simulink model "PID"  (R2021b)
settings: Solver=VariableStepAuto  StartTime=0.0  StopTime=10.0  RelTol=1e-3
settings Model: Creator=Studenci  LastModifiedBy=Studenci

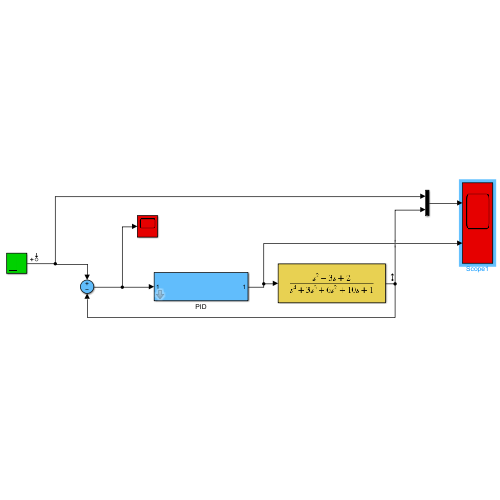
[thumbnail: Simulink's stored preview of the top-level diagram]
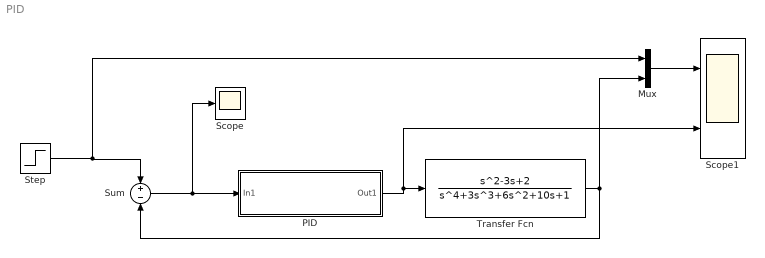
== system PID ==
  Mux : Mux  Inputs=2
  PID : Subsystem  mask{Kp=1.5288, Ki=0.4312, Kd=1.3550}
      mask prompts: Kp "Kp ="; Ki "Ki ="; Kd "Kd ="
  Scope : Scope
  Scope1 : Scope  NumInputPorts=2
  Step : Step  Time=0  SampleTime=0
  Sum : Sum  Inputs=+-
  Transfer Fcn : TransferFcn  Numerator=[1 -3 2]  Denominator=[1 3 6 10 1]
  wires:
  Step/1 -> Sum/1, Mux/1
  Sum/1 -> Scope/1, PID/1(In1)
  Mux/1 -> Scope1/1
  PID/1(Out1) -> Scope1/2, Transfer Fcn/1
  Transfer Fcn/1 -> Mux/2, Sum/2

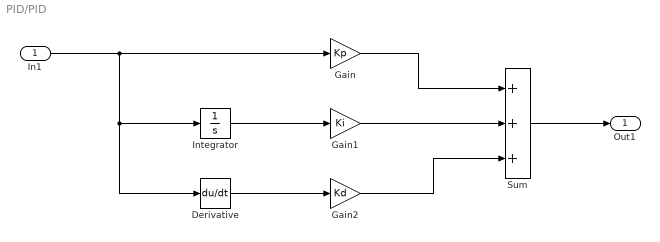
== system PID/PID ==
  In1 : Inport
  Derivative : Derivative
  Gain : Gain  Gain=Kp
  Gain1 : Gain  Gain=Ki
  Gain2 : Gain  Gain=Kd
  Integrator : Integrator
  Sum : Sum  Inputs=+++
  Out1 : Outport
  wires:
  Sum/1 -> Out1/1
  In1/1 -> Derivative/1, Integrator/1, Gain/1
  Gain/1 -> Sum/1
  Integrator/1 -> Gain1/1
  Gain1/1 -> Sum/2
  Gain2/1 -> Sum/3
  Derivative/1 -> Gain2/1
